simulink model "lin_maglev"  (R2025a)
settings: Solver=VariableStepAuto  StartTime=0.0  StopTime=1  RelTol=1e-3
values from neighbouring files (symbols this model uses):
  B = zeros(n, 1)    [GetLinModFtxu.m]
  C = tf(num, den)    [simulate.m]
  D = zeros(length(B), 1)    [simulate.m]
  den = [1 100]    [simulate.m]
  k = 2.9626e-4    (= 0.00029626)    [rhs.m]    (also in simulate.m = -162.15)
  num = [1 30]    [simulate.m]
  r = [.001; 0; 0]    [simulate.m]
  xs = [0.025;0;0.25;]    [simulate.m]
undefined symbols (not defined in the file or in its folder): A
settings Model: Creator=quintenpienaar  LastModifiedBy=quintenpienaar
settings DataIOCC: SaveOutput=off  SignalLogging=off  DSMLogging=off  SaveTime=off  ReturnWorkspaceOutputs=off

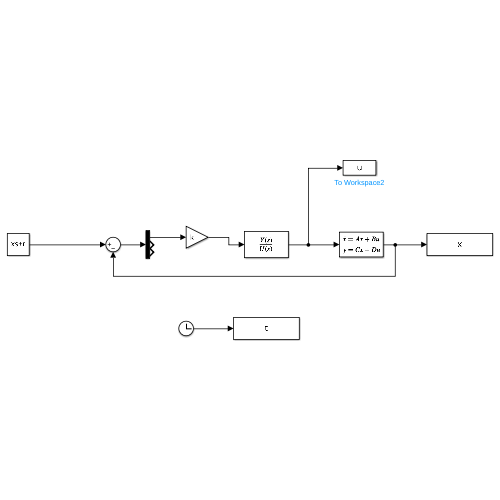
[thumbnail: Simulink's stored preview of the top-level diagram]
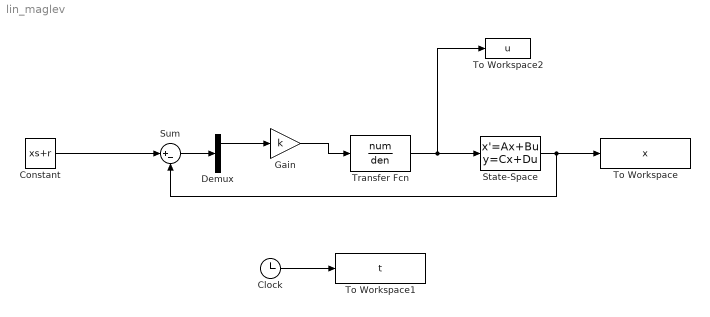
== system lin_maglev ==
  Clock : Clock
  Constant : Constant  Value=xs+r
  Demux : Demux  Outputs=3
  Gain : Gain  Gain=k
  State-Space : StateSpace  A=A  B=B  C=C  D=D  InitialCondition=0
  Sum : Sum  Inputs=|+-
  To Workspace : ToWorkspace  VariableName=x  SampleTime=-1
      settings: Save2DSignal=2-D array (concatenate along first dimension)
  To Workspace1 : ToWorkspace  VariableName=t  SampleTime=-1
      settings: Save2DSignal=2-D array (concatenate along first dimension)
  To Workspace2 : ToWorkspace  VariableName=u  SampleTime=-1
      settings: Save2DSignal=2-D array (concatenate along first dimension)
  Transfer Fcn : TransferFcn  Numerator=num  Denominator=den
  wires:
  Constant/1 -> Sum/1
  Clock/1 -> To Workspace1/1
  State-Space/1 -> Sum/2, To Workspace/1
  Transfer Fcn/1 -> To Workspace2/1, State-Space/1
  Sum/1 -> Demux/1
  Demux/1 -> Gain/1
  Gain/1 -> Transfer Fcn/1
